simulink model "Roadsense_SemanticMapFusion"  (R2025b)
settings: Solver=FixedStepDiscrete  StartTime=0.0  StopTime=1.0  FixedStep=RsTsBase  RelTol=1e-3
undefined symbols (not defined in the file or in its folder): RsGridCols, RsGridRows, RsMaxPredictionModes, RsMaxTracks, RsPredictionSteps, RsSemanticOutputHeight, RsSemanticOutputWidth, RsTsPlanning
settings Model: DataDictionary=Roadsense_Data.sldd  Creator=ragur  LastModifiedBy=ragur

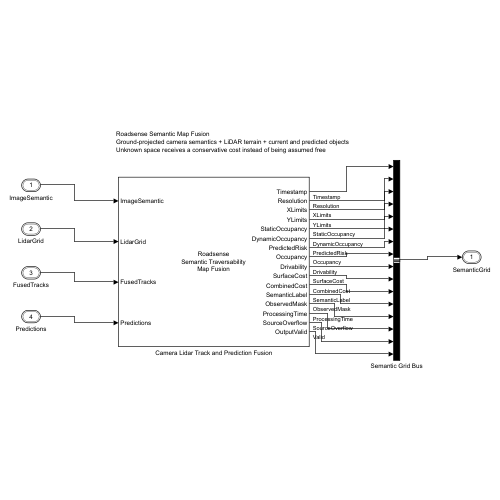
[thumbnail: Simulink's stored preview of the top-level diagram]
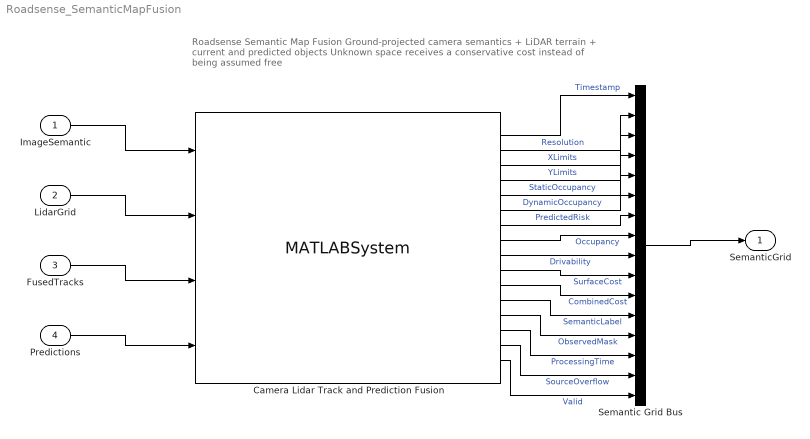
== system Roadsense_SemanticMapFusion ==
  note: Roadsense Semantic Map Fusion
      | Ground-projected camera semantics + LiDAR terrain + current and predicted objects
      | Unknown space receives a conservative cost instead of being assumed free
  ImageSemantic : Inport  OutDataTypeStr=Bus: RsImageSemanticBus  PortDimensions=1  SampleTime=RsTsPlanning
  LidarGrid : Inport  Port=2  OutDataTypeStr=Bus: RsLidarGridEvidenceBus  PortDimensions=1  SampleTime=RsTsPlanning
  FusedTracks : Inport  Port=3  OutDataTypeStr=Bus: RsFusedTrackListBus  PortDimensions=1  SampleTime=RsTsPlanning
  Predictions : Inport  Port=4  OutDataTypeStr=Bus: RsMotionPredictionListBus  PortDimensions=1  SampleTime=RsTsPlanning
  Camera Lidar Track and Prediction Fusion : MATLABSystem  System=RoadsenseSemanticMapFusionSystem  GridRows=double(RsGridRows)  GridCols=double(RsGridCols)  SemanticRows=double(RsSemanticOutputHeight)  SemanticCols=double(RsSemanticOutputWidth)  MaxTracks=double(RsMaxTracks)  MaxModes=double(RsMaxPredictionModes)  PredictionSteps=double(RsPredictionSteps)  GridResolution=RsGridResolution  GridXLimits=RsGridXLimits  GridYLimits=RsGridYLimits  CameraFocalLength=RsCameraFocalLength  CameraPrincipalPoint=RsCameraPrincipalPoint  CameraHeight=RsCameraHeight  CameraPitchDown=RsCameraPitchDown  UnknownDrivability=RsMapUnknownDrivability  CameraMinConfidence=RsMapCameraMinConfidence  CurrentSafetyMargin=RsMapCurrentSafetyMargin  MaximumCurrentInflation=RsMapMaximumCurrentInflation  PredictionSigma=RsMapPredictionSigma  MaximumPredictionRadius=RsMapMaximumPredictionRadius  PredictionTimeDecay=RsMapPredictionTimeDecay  PotholeThreshold=RsMapPotholeThreshold  SimulateUsing=Interpreted execution
      mask Type: RoadsenseSemanticMapFusionSystem
  Semantic Grid Bus : BusCreator  Inputs=16  OutDataTypeStr=Bus: RsSemanticGridBus
  SemanticGrid : Outport  OutDataTypeStr=Bus: RsSemanticGridBus
  wires:
  ImageSemantic/1 -> Camera Lidar Track and Prediction Fusion/1
  LidarGrid/1 -> Camera Lidar Track and Prediction Fusion/2
  FusedTracks/1 -> Camera Lidar Track and Prediction Fusion/3
  Predictions/1 -> Camera Lidar Track and Prediction Fusion/4
  Camera Lidar Track and Prediction Fusion/1 -> Semantic Grid Bus/1  "Timestamp"
  Camera Lidar Track and Prediction Fusion/2 -> Semantic Grid Bus/2  "Resolution"
  Camera Lidar Track and Prediction Fusion/3 -> Semantic Grid Bus/3  "XLimits"
  Camera Lidar Track and Prediction Fusion/4 -> Semantic Grid Bus/4  "YLimits"
  Camera Lidar Track and Prediction Fusion/5 -> Semantic Grid Bus/5  "StaticOccupancy"
  Camera Lidar Track and Prediction Fusion/6 -> Semantic Grid Bus/6  "DynamicOccupancy"
  Camera Lidar Track and Prediction Fusion/7 -> Semantic Grid Bus/7  "PredictedRisk"
  Camera Lidar Track and Prediction Fusion/8 -> Semantic Grid Bus/8  "Occupancy"
  Camera Lidar Track and Prediction Fusion/9 -> Semantic Grid Bus/9  "Drivability"
  Camera Lidar Track and Prediction Fusion/10 -> Semantic Grid Bus/10  "SurfaceCost"
  Camera Lidar Track and Prediction Fusion/11 -> Semantic Grid Bus/11  "CombinedCost"
  Camera Lidar Track and Prediction Fusion/12 -> Semantic Grid Bus/12  "SemanticLabel"
  Camera Lidar Track and Prediction Fusion/13 -> Semantic Grid Bus/13  "ObservedMask"
  Camera Lidar Track and Prediction Fusion/14 -> Semantic Grid Bus/14  "ProcessingTime"
  Camera Lidar Track and Prediction Fusion/15 -> Semantic Grid Bus/15  "SourceOverflow"
  Camera Lidar Track and Prediction Fusion/16 -> Semantic Grid Bus/16  "Valid"
  Semantic Grid Bus/1 -> SemanticGrid/1
